simulink model "astrobee_linear_pos_OL"  (R2015b)
settings: Solver=ode3  StartTime=0.0  StopTime=60  FixedStep=.01  RelTol=1e-3
libraries: astrobee_linear_pos_ctl_lib x1
settings Model: Creator=jfusco1  LastModifiedBy=jfusco1
settings DataIOCC: SaveFormat=Array
settings OptimizationCC: DefaultParameterBehavior=Inlined  BufferReuse=off
settings DebuggingCC: InitInArrayFormatMsg=none
settings HardwareCC: ProdBitPerPointer=32  ProdLargestAtomicFloat=None  ProdIntDivRoundTo=Undefined  ProdEndianess=Unspecified  ProdWordSize=32  ProdHWDeviceType=32-bit Generic
settings GRTTargetCC: GeneratePreprocessorConditionals=Disable all
settings ConfigComp: CovModelRefEnable=Off

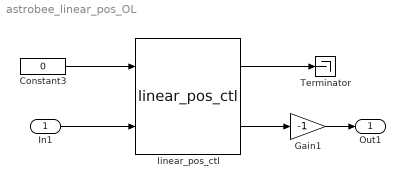
== system astrobee_linear_pos_OL ==
  In1 : Inport  PortDimensions=3
  Constant3 : Constant  Value=0
  Gain1 : Gain  Gain=-1
  Terminator : Terminator
  linear_pos_ctl : astrobee_linear_pos_ctl_lib/linear_pos_ctl
  Out1 : Outport
  wires:
  Constant3/1 -> linear_pos_ctl/1
  linear_pos_ctl/2 -> Gain1/1
  Gain1/1 -> Out1/1
  In1/1 -> linear_pos_ctl/2
  linear_pos_ctl/1 -> Terminator/1
